simulink model "Tractive_System_model"  (R2025b)
settings: Solver=ode15s  StartTime=0  StopTime=169.89  MaxStep=1e-3  RelTol=1e-3  AbsTol=1e-6
PreLoadFcn:
  | vehicleData
undefined symbols (not defined in the file): FL, FR, RL, RR, vehicle
libraries: batteryecm_lib x281, fl_lib x86, nesl_utility x54, ee_lib x16, sdl_lib x10, SimscapeFluids_lib x3, BatteryEstimators x2, simulink x1, slpidlib x1, autolibshared x1, eePmsmFieldOrientedControl x1
(part 1 of 26)
settings Model: SimulationMode=accelerator  PacingRate=0.002200  Creator=muizz  LastModifiedBy=muizz
settings SolverCC: AutoScaleAbsTol=off  MaxConsecutiveMinStep=10000  ZeroCrossAlgorithm=Adaptive
settings DebuggingCC: AlgebraicLoopMsg=none  IgnoredZcDiagnostic=none

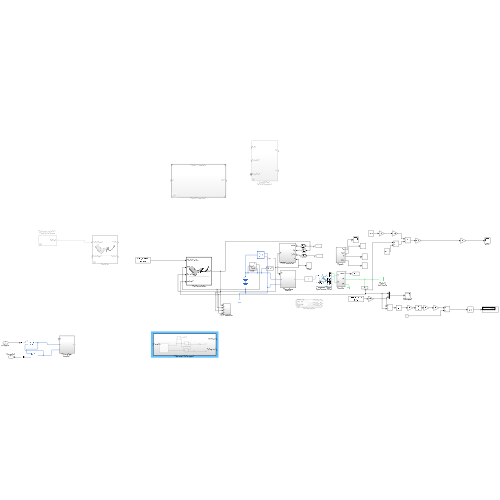
[thumbnail: Simulink's stored preview of the top-level diagram]
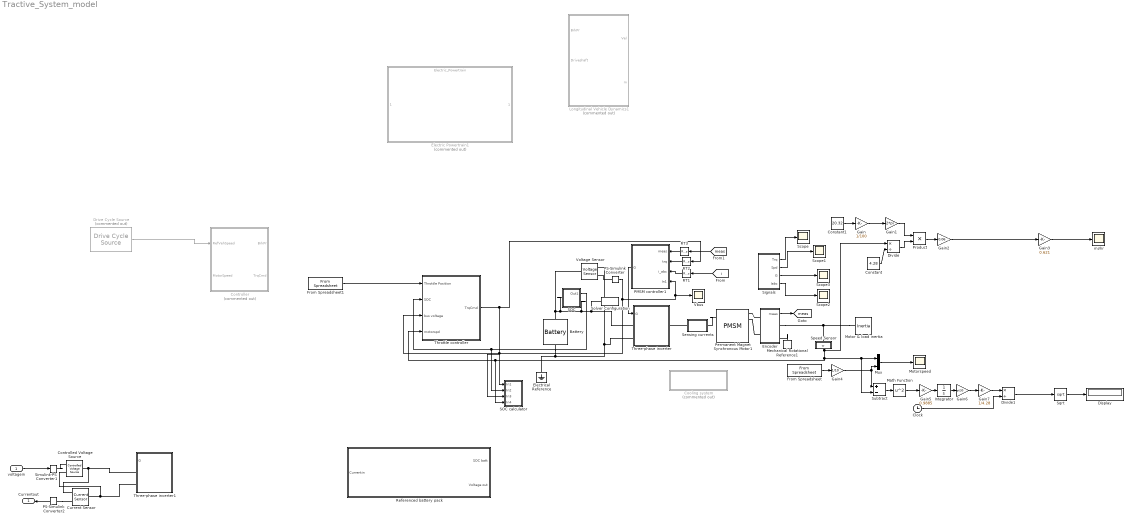
== system Tractive_System_model ==
  voltagein : Inport
  Battery : batteryecm_lib/Battery  Vnom=450 V  prm_dir=1  R1_dis=2 Ohm  R1_ch=2 Ohm  R1=0.001 Ohm  prm_AH=1  AH=14000 hr*A  V1=470 V  AH1=5000 hr*A  prm_R2=1  R2=inf Ohm  Tmeas=298.15 K  charge_measurement_port=simscape.enum.battery.enable.no  prm_dyn=1  Rp1=0.005 Ohm  tau1=30 s  Rp2=0.005 Ohm  tau2=30 s  Rp3=0.005 Ohm  tau3=30 s  Rp4=0.005 Ohm  tau4=30 s  Rp5=0.005 Ohm  tau5=30 s  prm_fade=1  N_fade=100  AH_fade=45 hr*A  R1_fade=2.02 Ohm  R1_ch_fade=2.02 Ohm  V1_fade=10.35 V  prm_age=1  prm_age_OCV=1  OCV_age=0.9  SOC_age=60  Tmeas_age=298.15 K  delta_time_age_vec=[0] d  temperature_age_vec=[273] K  OCV_scaling_age=2.2134e6  OCV_offset_age=1.632e6  temp_exp_age=0.515833569 V  t_exp_age=0.75  Vnom_T2=12 V  R1_T2=2.2 Ohm  R1_T2_dis=2.2 Ohm  R1_T2_ch=2.2 Ohm  V1_T2=11.4 V  R2_T2=2200 Ohm  Rp1_T2=0.005 Ohm  tau1_T2=30 s  Rp2_T2=0.005 Ohm  tau2_T2=30 s  Rp3_T2=0.005 Ohm  tau3_T2=30 s  Rp4_T2=0.005 Ohm  tau4_T2=30 s  Rp5_T2=0.005 Ohm  tau5_T2=30 s  Tmeas2=273.15 K  thermal_port=simscape.enum.thermaleffects.omit  thermal_mass=30000 J/K  i_specify=off  i_priority=None  i=0 A  i_nominal_specify=off  i_nominal_value=1  i_nominal_unit=A  v_specify=off  v_priority=None  v=0 V  v_nominal_specify=off  v_nominal_value=1  v_nominal_unit=V  charge_specify=on  charge_priority=High  charge=7000 hr*A  charge_nominal_specify=off  charge_nominal_value=1  charge_nominal_unit=A*hr  num_cycles_specify=off  num_cycles_priority=High  num_cycles=0  num_cycles_nominal_specify=off  num_cycles_nominal_value=1  num_cycles_nominal_unit=1  temperature_specify=off  temperature_priority=High  temperature=298.15 K  temperature_nominal_specify=off  temperature_nominal_value=1  temperature_nominal_unit=K
  Clock : Clock
  Constant : Constant  Value=4.28
  Constant1 : Constant  Value=20.32
  Controlled Voltage Source : fl_lib/Electrical/Electrical Sources/Controlled Voltage Source
  Controller : Subsystem  Commented=on  TreatAsAtomicUnit=on
      mask Display: image('Images/brakeThrottle.png'); % Use "Edit Image" on toolstrip to change.
  Cooling system : Subsystem  Commented=on
  Current Sensor : fl_lib/Electrical/Electrical Sensors/Current Sensor
  Display : Display
  Divide : Product  Inputs=*/
  Divide1 : Product  Inputs=*/
  Drive Cycle Source : autolibshared/Drive Cycle Source  Commented=on  cycleVar=Workspace variable  wsVar=fsdCycle  fileVar=cycleFTP75.mat  tfinal=""  cycleRepeat=on  outAccPort=off  outGearPort=off  gearList=No gear data  t_wot1=5  xdot_woto=0  xdot_wot1=30  t_wot2=20  xdot_wot2=0  t_wotend=30  srcUnit=m/s  outUnit=km/h  srcAccUnit=m/s/s  outAccUnit=m/s^2  dt=0  aMode=1  faultOption=off  velBnd=2  velBndUnit=mph  inUnit=m/s  timeBnd=1  failOption=off  stopSim=off  maxFaultCnt=10  maxFaultTime=2  maxTotFaultTime=15  traceOption=off  dtTrace=1  traceWindow=10  lastDCname=Custom Data Set  lastOutUnit=mph  lastDT=0  lastTB=1  lastSB=2  forceCalcBound=off
  Electric Powertrain1 : ModelReference  Commented=on  ModelNameDialog=Electric_Powertrain.slx  SimulationMode=Normal  ModelReferenceVersion=1.80
  Electrical Reference : fl_lib/Electrical/Electrical Elements/Electrical Reference
  Encoder : Subsystem
  From Spreadsheet : FromSpreadsheet  FileName=E25_Run1.xls  SheetName=RPM
  From Spreadsheet1 : FromSpreadsheet  FileName=E25_Run1.xls  SheetName=Throttle
  Gain : Gain  Gain=1/100
  Gain1 : Gain  Gain=2*pi
  Gain2 : Gain  Gain=0.06
  Gain3 : Gain  Gain=0.621
  Gain4 : Gain  Gain=1/10
  Gain5 : Gain  Gain=0.9885
  Gain6 : Gain  Gain=pi/30
  Gain7 : Gain  Gain=1/4.28
  Integrator : Integrator
  Longitudinal Vehicle Dynamics1 : Subsystem  Commented=on
  Math Function : Math  Operator=square
  Mechanical Rotational Reference1 : fl_lib/Mechanical/Rotational Elements/Mechanical Rotational Reference
  Motor & load inertia : fl_lib/Mechanical/Rotational Elements/Inertia  inertia=1.0116 kg*m^2  num_ports=foundation.enum.numPorts2.one  w_specify=on  w_priority=High  w=0 rpm  w_nominal_specify=off  w_nominal_value=1  w_nominal_unit=rad/s  t_specify=off  t_priority=High  t=0 N*m  t_nominal_specify=off  t_nominal_value=1  t_nominal_unit=N*m
  Motorspeed : Scope
      settings: ActiveDisplayYMinimum=-689.17048059754359  ActiveDisplayYMaximum=5992.5343253778938  DataLoggingVariableName=ScopeData5
  Mux : Mux  Inputs=2
  PMSM controller1 : Subsystem
  PS-Simulink Converter : nesl_utility/PS-Simulink Converter  PhysicalDomain=network_engine_domain  SubClassName=ps_output  LeftPortType=input  RightPortType=output  PseudoPeriodic=off  Frequencies=[]  VectorFormat=inherit  Unit=inherit  AffineConversion=off
  PS-Simulink Converter2 : nesl_utility/PS-Simulink Converter  PhysicalDomain=network_engine_domain  SubClassName=ps_output  LeftPortType=input  RightPortType=output  PseudoPeriodic=off  Frequencies=[]  VectorFormat=inherit  Unit=inherit  AffineConversion=off
  Permanent Magnet Synchronous Motor1 : ee_lib/Electromechanical/Permanent Magnet/PMSM  port_option=ee.enum.threePhasePort.composite  winding_type=ee.enum.statorconnection.wye  machine_param=ee.enum.pmsm.parameterization.constant  nPolePairs=10  pmflux_param=ee.enum.pmflux.fluxlinkage  pm_flux_linkage=0.04 Wb  torque_constant=0.18 N*m/A  back_emf_constant=0.18 V/(rad/s)  stator_param=ee.enum.statorparam.LdLqL0  Ld=1.25e-4 H  Lq=1.3e-4 H  idVec=[-200, 0, 200] A  iqVec=[-200, 0, 200] A  LdMatrix=0.0002 * ones(3, 3) H  LqMatrix=0.0002 * ones(3, 3) H  PmMatrix=0.1 * ones(3, 3) Wb  ktMatrix=0.18 * ones(3, 3) N*m/A  keMatrix=0.18 * ones(3, 3) V/(rad/s)  L0=L0 H  Ls=0.0002 H  Lm=0.00002 H  Ms=0.00002 H  Rs=0.012 Ohm  zero_sequence=ee.enum.park.zerosequence.exclude  axes_param=ee.enum.rotorangle.qaxis  loss_param=ee.enum.ironloss.none  losses_oc=[0, 0, 0] W  losses_sc=[0, 0, 0] W  f_losses=60 Hz  Isc_losses=95 A  J=0 kg*m^2  lam=0 N*m/(rad/s)  i_d_specify=off  i_d_priority=None  i_d=0 A  i_d_nominal_specify=off  i_d_nominal_value=1  i_d_nominal_unit=A  i_q_specify=off  i_q_priority=None  i_q=0 A  i_q_nominal_specify=off  i_q_nominal_value=1  i_q_nominal_unit=A  torque_specify=off  torque_priority=None  torque=0 N*m  torque_nominal_specify=off  torque_nominal_value=1  torque_nominal_unit=N*m  angular_velocity_specify=on  angular_velocity_priority=None  angular_velocity=0 rpm  angular_velocity_nominal_specify=off  angular_velocity_nominal_value=1  angular_velocity_nominal_unit=rpm  angular_position_specify=on  angular_position_priority=High  angular_position=0 rad  angular_position_nominal_specify=off  angular_position_nominal_value=1  angular_position_nominal_unit=deg  alpha=3.93e-3 1/K  alpha_flux=-0.001 1/K  Tmeas=298.15 K  stator_thermal_mass=100 J/K  rotor_thermal_mass=200 J/K  Rm_percent_rotor=90  Rd_percent_rotor=30  temperatureA_specify=off  temperatureA_priority=High  temperatureA=25 degC  temperatureA_nominal_specify=off  temperatureA_nominal_value=1  temperatureA_nominal_unit=degC  temperatureB_specify=off  temperatureB_priority=High  temperatureB=25 degC  temperatureB_nominal_specify=off  temperatureB_nominal_value=1  temperatureB_nominal_unit=degC  temperatureC_specify=off  temperatureC_priority=High  temperatureC=25 degC  temperatureC_nominal_specify=off  temperatureC_nominal_value=1  temperatureC_nominal_unit=degC  temperatureR_specify=off  temperatureR_priority=High  temperatureR=25 degC  temperatureR_nominal_specify=off  temperatureR_nominal_value=1  temperatureR_nominal_unit=degC
      settings: InternalSimscapePortConfiguration="{\"Bottom\":[],\"Left\":[{\"id\":\"N\",\"label\":\"~\",\"type\":\"foundation.electrical.three_phase\"},{\"id\":\"HR\",\"label\":\"HR\",\"type\":\"foundation.thermal.thermal\"}],\"Right\":[{\"id\":\"R\",\"label\":\"R\",\"type\":\"foundation.mechanical.rotational.rotational\"},{\"id\":\"C\",\"label\":\"C\",\"type\":\"foundation.mechanical.rotational.rotational\"},{\"id\":\"HA\",\"label\":\"HA\",\"type\":\"foundation.thermal.thermal\"},{\"id\":\"HB\",\"label\":\"HB\",\"type\":\"foundation.thermal.thermal\"},{\"id\":\"HC\",\"label\":\"HC\",\"type\":\"foundation.thermal.thermal\"}],\"Top\":[]}"
  Product : Product
  RT1 : RateTransition  OutPortSampleTime=1e-5
  RT2 : RateTransition  OutPortSampleTime=1e-5
  RT3 : RateTransition  OutPortSampleTime=1e-5
  "Referenced battery pack " : Subsystem  TreatAsAtomicUnit=on
  SOC : Subsystem
  SOC calculator : Subsystem
  Scope{,1..3} (4 alike) : Scope
      Scope settings: ActiveDisplayYMinimum=-50.625253953054461  ActiveDisplayYMaximum=50.62524512492179  DataLoggingVariableName=ScopeData6
      Scope1 settings: ActiveDisplayYMinimum=-1907.899738969727  ActiveDisplayYMaximum=6138.7110691558973  DataLoggingVariableName=ScopeData7
      Scope2 settings: ActiveDisplayYMinimum=-181.90652911018958  ActiveDisplayYMaximum=169.90814228402508  DataLoggingVariableName=ScopeData8
      Scope3 settings: ActiveDisplayYMinimum=-1  ActiveDisplayYMaximum=1  DataLoggingVariableName=ScopeData9
  Sensing currents : Subsystem
      mask Display: disp('i')
  "Signals " : Subsystem
  Simulink-PS Converter1 : nesl_utility/Simulink-PS Converter  PhysicalDomain=network_engine_domain  SubClassName=ps_input  LeftPortType=input  RightPortType=output  PseudoPeriodic=off  Frequencies=[]  NoiseDistribution=none  NoiseParameters=[]  Unit=1  AffineConversion=off  FilteringAndDerivatives=provide  SimscapeFilterOrder=1  InputFilterTimeConstant=0.001  UdotUserProvided=0
  Solver Configuration : nesl_utility/Solver Configuration  PhysicalDomain=network_engine_domain  SubClassName=solver  LeftPortType=input  RightPortType=generic  Tones=[]  Harmonics=[]  SimulateNoise=off  Profile=off  UseLocalSampling=off  EnableSwitchedLinearOptims=on  FrequencyDomain=off  UseCCode=off  RelTol=0.001  AbsTol=1e-06  MinStep=1e-09  ToWorkspace=off  RevertToSquareIcSolve=off  NumHomotopyIterations=100  PhasorMode=off  PhasorModeNumHarmonics=1  ConsistencySolver=NEWTON_FTOL  IndexReductionMethod=DerivativeReplacement  DoDC=off  ResidualTolerance=1e-9  ConsistencyTolSource=GLOBAL  ConsistencyAbsTol=0.001  ConsistencyRelTol=0.001  ConsistencyTolFactor=0.001  UseLocalSolver=on  LocalSolverChoice=NE_PARTITIONING_ADVANCER  ResolveIndetEquations=on  FunctionEvalNumThread=1  LocalSolverSampleTime=1e-5  DoFixedCost=off  MaxNonlinIter=4  MaxModeIter=2  ComputeImpulses=off  ImpulseIterations=2  LinearAlgebra=auto  LinearAlgebraNumThread=0  EquationFormulation=NE_TIME_EF  DelaysMemoryBudget=1024  AutomaticFiltering=on  FilteringTimeConstant=0.001  PartitionStorageMethod=AS_NEEDED  PartitionMemoryBudget=1024  PartitionMethod=FAST  MultibodyUseLocalSolver=off  MultibodyLocalSolverChoice=ODE1  MultibodyLocalSolverSampleTime=0.001
  Speed Sensor : Subsystem
      mask Display: disp('w')
  Sqrt : Sqrt
  Subtract : Sum  Inputs=+-
  Three-phase inverter : Subsystem
  Three-phase inverter1 : Subsystem
  Throttle controller : Subsystem  TreatAsAtomicUnit=on
      mask Display: image('Images/brakeThrottle.png'); % Use "Edit Image" on toolstrip to change.
  Vbus : Scope
      settings: ActiveDisplayYMinimum=403.93858192794437  ActiveDisplayYMaximum=455.46174198734315  DataLoggingVariableName=ScopeData13
  Voltage Sensor : fl_lib/Electrical/Electrical Sensors/Voltage Sensor
  mi/hr : Scope
      settings: ActiveDisplayYMinimum=-2.4921742496498496  ActiveDisplayYMaximum=69.067219320709555  DataLoggingVariableName=ScopeData4
  Currentout : Outport
  tag scope: meas=global
  wires:
  Drive Cycle Source/1 -> Controller/1(RefVehSpeed)
  "Signals "/1(Trq) -> Scope/1
  Gain/1 -> Gain1/1
  "Signals "/4(Iabc) -> Scope2/1
  "Signals "/3(G) -> Scope3/1
  "Signals "/2(Spd) -> Scope1/1
  Constant/1 -> Divide/2
  Divide/1 -> Product/2
  Constant1/1 -> Gain/1
  PS-Simulink Converter/1 -> SOC calculator/3(In3), Throttle controller/3(bus voltage), Vbus/1, PMSM controller1/4(In1)
  Speed Sensor/1(w) -> SOC calculator/4(In4), Throttle controller/4(motorspd), Mux/1, Subtract/2, Divide/1
  Gain1/1 -> Product/1
  Product/1 -> Gain2/1
  Encoder/1(meas) -> [meas]
  Gain3/1 -> mi/hr/1
  From Spreadsheet1/1 -> Throttle controller/1(Throttle Position)
  SOC/1(Out1) -> SOC calculator/2(In2), Throttle controller/2(SOC)
  Throttle controller/1(TrqCmd) -> SOC calculator/1(In1), RT2/1
  RT1/1 -> PMSM controller1/3(i_abc)
  RT3/1 -> PMSM controller1/1(meas)
  [i] -> RT1/1
  [meas] -> RT3/1
  PMSM controller1/1(G) -> Three-phase inverter/1(G)
  RT2/1 -> PMSM controller1/2(trq)
  Gain2/1 -> Gain3/1
  Mux/1 -> Motorspeed/1
  Gain4/1 -> Subtract/1, Mux/2
  From Spreadsheet/1 -> Gain4/1
  Subtract/1 -> Math Function/1
  Math Function/1 -> Gain5/1
  Divide1/1 -> Sqrt/1
  Integrator/1 -> Gain6/1
  Sqrt/1 -> Display/1
  Clock/1 -> Divide1/2
  Gain5/1 -> Integrator/1
  Gain6/1 -> Gain7/1
  Gain7/1 -> Divide1/1
  PS-Simulink Converter2/1 -> Currentout/1
  voltagein/1 -> Simulink-PS Converter1/1
  connections:
  Voltage Sensor/RConn2 -- Electrical Reference/LConn1 -- Battery/RConn1 -- Three-phase inverter/LConn2
  Motor & load inertia/LConn1 -- Encoder/RConn1 -- Speed Sensor/LConn1
  Solver Configuration/RConn1 -- SOC/RConn1 -- Voltage Sensor/LConn1 -- Battery/LConn1 -- SOC/LConn1 -- Three-phase inverter/LConn1
  Encoder/LConn1 -- Permanent Magnet Synchronous Motor1/RConn1
  PS-Simulink Converter/LConn1 -- Voltage Sensor/RConn1
  Permanent Magnet Synchronous Motor1/LConn1 -- Sensing currents/RConn1
  Encoder/LConn2 -- Permanent Magnet Synchronous Motor1/RConn2
  Sensing currents/LConn1 -- Three-phase inverter/RConn1
  Mechanical Rotational Reference1/LConn1 -- Encoder/RConn2
  Three-phase inverter1/LConn2 -- Controlled Voltage Source/RConn2 -- Current Sensor/LConn1
  Controlled Voltage Source/LConn1 -- Current Sensor/RConn2 -- Three-phase inverter1/LConn1
  PS-Simulink Converter2/LConn1 -- Current Sensor/RConn1
  Simulink-PS Converter1/RConn1 -- Controlled Voltage Source/RConn1

== system Tractive_System_model/Controller ==
  RefVehSpeed : Inport
  MotorSpeed : Inport  Port=2
  Control : Subsystem
  Motor Speed Reference : Subsystem
  Motor spd : Scope
      settings: ActiveDisplayYMinimum=-557.16498453715531  ActiveDisplayYMaximum=5014.4848608343991  DataLoggingVariableName=ScopeData3
  BrkPr : Outport
  TrqCmd : Outport  Port=2
  tag scope: Ref=global
  wires:
  RefVehSpeed/1 -> [Ref], Motor Speed Reference/1(VehSpd)
  MotorSpeed/1 -> Control/1(In1)
  Motor Speed Reference/1(MotorSpdRef) -> Motor spd/1, Control/2(Motor Speed Ref)  "Motor Speed Ref"
  Control/1(Cal Pressure) -> BrkPr/1
  Control/2(MotCmdTrq) -> TrqCmd/1  "Motor Speed"

== system Tractive_System_model/Cooling system ==
  Ambient Temperature : fl_lib/Physical Signals/Sources/PS Constant  constant=300.15 K
  "Cooling system " : Subsystem
  Subsystem1 : Subsystem
  Temperature Source : fl_lib/Thermal/Thermal Sources/Controlled Temperature Source
  Thermal Reference : fl_lib/Thermal/Thermal Elements/Thermal Reference
  Thermal model : Subsystem  Tag=PublishSubsystem
  ARMS_IN : PMIOPort  Side=Left
  VDC_IN : PMIOPort  Port=2  Side=Left
  Winding C : PMIOPort  Port=3  Side=Right
  Winding B : PMIOPort  Port=4  Side=Right
  Winding A : PMIOPort  Port=5  Side=Right
  Pressure : PMIOPort  Port=6  Side=Left
  Rotor : PMIOPort  Port=7  Side=Left
  connections:
  Subsystem1/LConn2 -- VDC_IN/RConn1
  "Cooling system "/LConn1 -- Pressure/RConn1
  Thermal model/RConn2 -- Winding B/RConn1
  Temperature Source/RConn2 -- Thermal Reference/LConn1
  Thermal model/RConn3 -- Winding A/RConn1
  Temperature Source/LConn1 -- Thermal model/LConn2
  Thermal model/LConn1 -- Rotor/RConn1 -- "Cooling system "/RConn2
  Ambient Temperature/RConn1 -- Temperature Source/RConn1
  Subsystem1/RConn1 -- "Cooling system "/RConn1
  Thermal model/RConn1 -- Winding C/RConn1
  Subsystem1/LConn1 -- ARMS_IN/RConn1

== system Tractive_System_model/Encoder ==
  Ideal Rotational Motion Sensor : fl_lib/Mechanical/Mechanical Sensors/Ideal Rotational Motion Sensor  reference=foundation.enum.MeasurementReference.difference  acceleration_port=false  velocity_port=true  position_port=true  wrap_angle=simscape.enum.onoff.off  offset=0 deg
  Ideal Torque Sensor : fl_lib/Mechanical/Mechanical Sensors/Ideal Torque Sensor
  Mux : Mux  Inputs=2
  PS-Simulink Converter : nesl_utility/PS-Simulink Converter  PhysicalDomain=network_engine_domain  SubClassName=ps_output  LeftPortType=input  RightPortType=output  PseudoPeriodic=off  Frequencies=[]  VectorFormat=1-D array  Unit=rad/s  AffineConversion=off
  PS-Simulink Converter1 : nesl_utility/PS-Simulink Converter  PhysicalDomain=network_engine_domain  SubClassName=ps_output  LeftPortType=input  RightPortType=output  PseudoPeriodic=off  Frequencies=[]  VectorFormat=1-D array  Unit=rad  AffineConversion=off
  PS-Simulink Converter2 : nesl_utility/PS-Simulink Converter  PhysicalDomain=network_engine_domain  SubClassName=ps_output  LeftPortType=input  RightPortType=output  PseudoPeriodic=off  Frequencies=[]  VectorFormat=1-D array  Unit=N*m  AffineConversion=off
  1L : PMIOPort  Side=Left
  2L : PMIOPort  Port=2  Side=Left
  1R : PMIOPort  Port=3  Side=Right
  2R : PMIOPort  Port=4  Side=Right
  meas : Outport  VectorParamsAs1DForOutWhenUnconnected=off
  tag scope: trqMotor=global, wMotor=global
  wires:
  PS-Simulink Converter2/1 -> [trqMotor]
  Mux/1 -> meas/1
  PS-Simulink Converter1/1 -> Mux/2
  PS-Simulink Converter/1 -> [wMotor], Mux/1
  connections:
  Ideal Torque Sensor/RConn2 -- PS-Simulink Converter2/LConn1
  1L/RConn1 -- Ideal Torque Sensor/LConn1
  2R/RConn1 -- 2L/RConn1 -- Ideal Rotational Motion Sensor/RConn1
  Ideal Rotational Motion Sensor/LConn1 -- 1R/RConn1 -- Ideal Torque Sensor/RConn1
  Ideal Rotational Motion Sensor/RConn2 -- PS-Simulink Converter/LConn1
  Ideal Rotational Motion Sensor/RConn3 -- PS-Simulink Converter1/LConn1

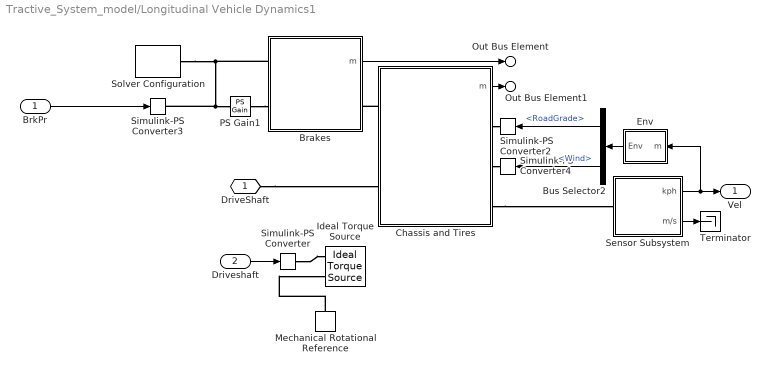
== system Tractive_System_model/Longitudinal Vehicle Dynamics1 ==
  BrkPr : Inport
  Driveshaft : Inport  Port=2
  Brakes : Subsystem
  Bus Selector2 : BusSelector  OutputSignals=RoadGrade,Wind
  Chassis and Tires : Subsystem
  Env : Subsystem
  Ideal Torque Source : fl_lib/Mechanical/Mechanical Sources/Ideal Torque Source
  Mechanical Rotational Reference : fl_lib/Mechanical/Rotational Elements/Mechanical Rotational Reference
  PS Gain1 : fl_lib/Physical Signals/Functions/PS Gain  gain=1
  Sensor Subsystem : Subsystem
  Simulink-PS Converter : nesl_utility/Simulink-PS Converter  PhysicalDomain=network_engine_domain  SubClassName=ps_input  LeftPortType=input  RightPortType=output  PseudoPeriodic=off  Frequencies=[]  NoiseDistribution=none  NoiseParameters=[]  Unit=N*m  AffineConversion=off  FilteringAndDerivatives=provide  SimscapeFilterOrder=1  InputFilterTimeConstant=0.001  UdotUserProvided=0
  Simulink-PS Converter2 : nesl_utility/Simulink-PS Converter  PhysicalDomain=network_engine_domain  SubClassName=ps_input  LeftPortType=input  RightPortType=output  PseudoPeriodic=off  Frequencies=[]  NoiseDistribution=none  NoiseParameters=[]  Unit=rad  AffineConversion=off  FilteringAndDerivatives=provide  SimscapeFilterOrder=1  InputFilterTimeConstant=0.001  UdotUserProvided=0
  Simulink-PS Converter3 : nesl_utility/Simulink-PS Converter  PhysicalDomain=network_engine_domain  SubClassName=ps_input  LeftPortType=input  RightPortType=output  PseudoPeriodic=off  Frequencies=[]  NoiseDistribution=none  NoiseParameters=[]  Unit=N/m^2  AffineConversion=off  FilteringAndDerivatives=provide  SimscapeFilterOrder=1  InputFilterTimeConstant=0.001  UdotUserProvided=0
  Simulink-PS Converter4 : nesl_utility/Simulink-PS Converter  PhysicalDomain=network_engine_domain  SubClassName=ps_input  LeftPortType=input  RightPortType=output  PseudoPeriodic=off  Frequencies=[]  NoiseDistribution=none  NoiseParameters=[]  Unit=m/s  AffineConversion=off  FilteringAndDerivatives=provide  SimscapeFilterOrder=1  InputFilterTimeConstant=0.001  UdotUserProvided=0
  Solver Configuration : nesl_utility/Solver Configuration  PhysicalDomain=network_engine_domain  SubClassName=solver  LeftPortType=input  RightPortType=generic  Tones=[]  Harmonics=[]  SimulateNoise=off  Profile=off  UseLocalSampling=off  EnableSwitchedLinearOptims=on  FrequencyDomain=off  UseCCode=off  RelTol=0.001  AbsTol=0.001  MinStep=1e-09  ToWorkspace=off  RevertToSquareIcSolve=off  NumHomotopyIterations=100  PhasorMode=off  PhasorModeNumHarmonics=1  ConsistencySolver=NEWTON_XTOL_AFTER_FTOL  IndexReductionMethod=DerivativeReplacement  DoDC=off  ResidualTolerance=1e-09  ConsistencyTolSource=GLOBAL  ConsistencyAbsTol=0.001  ConsistencyRelTol=0.001  ConsistencyTolFactor=0.001  UseLocalSolver=on  LocalSolverChoice=NE_BACKWARD_EULER_ADVANCER  ResolveIndetEquations=on  FunctionEvalNumThread=1  LocalSolverSampleTime=1e-4  DoFixedCost=off  MaxNonlinIter=3  MaxModeIter=2  ComputeImpulses=off  ImpulseIterations=2  LinearAlgebra=auto  LinearAlgebraNumThread=0  EquationFormulation=NE_TIME_EF  DelaysMemoryBudget=1024  AutomaticFiltering=on  FilteringTimeConstant=0.001  PartitionStorageMethod=AS_NEEDED  PartitionMemoryBudget=1024  PartitionMethod=ROBUST  MultibodyUseLocalSolver=off  MultibodyLocalSolverChoice=ODE1  MultibodyLocalSolverSampleTime=0.001
  Terminator : Terminator
  DriveShaft : PMIOPort  Side=Left
  Vel : Outport
  Out Bus Element : Outport  Port=2  PortName=m  Element=Brakes
  Out Bus Element1 : Outport  Port=2  PortName=m  Element=Chassis
  wires:
  Sensor Subsystem/1(kph) -> Vel/1, Env/1(m)
  Env/1(Env) -> Bus Selector2/1
  Bus Selector2/1 -> Simulink-PS Converter2/1  "<RoadGrade>"
  Bus Selector2/2 -> Simulink-PS Converter4/1  "<Wind>"
  BrkPr/1 -> Simulink-PS Converter3/1
  Sensor Subsystem/2(m/s) -> Terminator/1
  Brakes/1(m) -> Out Bus Element/1
  Chassis and Tires/1(m) -> Out Bus Element1/1
  Driveshaft/1 -> Simulink-PS Converter/1
  connections:
  Brakes/LConn1 -- Solver Configuration/RConn1 -- Simulink-PS Converter3/RConn1 -- PS Gain1/LConn1
  Chassis and Tires/RConn1 -- Simulink-PS Converter2/RConn1
  Chassis and Tires/RConn2 -- Simulink-PS Converter4/RConn1
  Chassis and Tires/LConn1 -- Brakes/RConn1
  Chassis and Tires/RConn3 -- Sensor Subsystem/LConn1
  PS Gain1/RConn1 -- Brakes/LConn2
  DriveShaft/RConn1 -- Chassis and Tires/LConn2
  Mechanical Rotational Reference/LConn1 -- Ideal Torque Source/RConn2
  Simulink-PS Converter/RConn1 -- Ideal Torque Source/RConn1

== system Tractive_System_model/PMSM controller1 ==
  meas : Inport
  trq : Inport  Port=2
  i_abc : Inport  Port=3
  In1 : Inport  Port=4
  Bus Selector : BusSelector  OutputSignals=iabc [A],Reference,TqRef [N*m]
  Demux1 : Demux  Outputs=2
  PMSM Field-Oriented Control : eePmsmFieldOrientedControl/PMSM Field-Oriented Control  winding_type=Wye-wound  CtrlMode=Torque control  Vnom=600  Pmax=80000  Tmax=150  p=10  Vdc_on=10  Ts=1e-5  Tsc=Tsc  CtrlType=PI control  Kp_w=60  Ki_w=300*2  Kv_w=1  Kaw_w=1000  RefType=Zero d-axis control  rpmVec=[0, 3000]  TqVec=[-100, 0, 100]  VdcVec=[300, 350]  PWMMode=SPWM: sinusoidal PWM  ModFactor=1  idMatrix=zeros(2,3,2)  iqMatrix=zeros(2,3,2)  psim=0.04  Ld=0.00024  Lq=0.00029  Rs=0.01  AxisAlignment=Q-axis  Kp_id=0.7854  Ki_id=75.4  Kaw_id=1000  Kp_iq=0.8168  Ki_iq=75.40  Kaw_iq=1000  AxisPrio=Q-axis  ActZC=off  ActFF=on  ParamTypeFF=Constant parameters  LdFF=1.25e-4  LqFF=1.3e-4  psimFF=0.04  idVect=[-200, 0, 200]  iqVect=[-200, 0, 200]  LdMatrix=0.0002 * ones(3, 3)  LqMatrix=0.0002 * ones(3, 3)  psimMatrix=0.04 * ones(3, 3)  CPWMMode=SPWM: sinusoidal PWM  fsw=10000
  G : Outport  VectorParamsAs1DForOutWhenUnconnected=off
  tag scope: G=global, iMotor=global, trqDemand=global, wDemand=global
  wires:
  PMSM Field-Oriented Control/1 -> G/1, [G]
  In1/1 -> PMSM Field-Oriented Control/5
  PMSM Field-Oriented Control/2 -> Bus Selector/1
  i_abc/1 -> PMSM Field-Oriented Control/2
  meas/1 -> Demux1/1
  Demux1/1 -> PMSM Field-Oriented Control/3
  Demux1/2 -> PMSM Field-Oriented Control/4
  Bus Selector/1 -> [iMotor]  "<iabc [A]>"
  Bus Selector/2 -> [wDemand]  "<Reference>"
  Bus Selector/3 -> [trqDemand]  "<TqRef [N*m]>"
  trq/1 -> PMSM Field-Oriented Control/1

== system Tractive_System_model/Referenced battery pack  ==
  Currentin : Inport
  Accumalator : Subsystem
  Controlled Current Source : fl_lib/Electrical/Electrical Sources/Controlled Current Source
  PS-Simulink Converter1 : nesl_utility/PS-Simulink Converter  PhysicalDomain=network_engine_domain  SubClassName=ps_output  LeftPortType=input  RightPortType=output  PseudoPeriodic=off  Frequencies=[]  VectorFormat=inherit  Unit=inherit  AffineConversion=off
  SOC1 : Subsystem
  Simulink-PS Converter : nesl_utility/Simulink-PS Converter  PhysicalDomain=network_engine_domain  SubClassName=ps_input  LeftPortType=input  RightPortType=output  PseudoPeriodic=off  Frequencies=[]  NoiseDistribution=none  NoiseParameters=[]  Unit=1  AffineConversion=off  FilteringAndDerivatives=provide  SimscapeFilterOrder=1  InputFilterTimeConstant=0.001  UdotUserProvided=0
  Voltage Sensor1 : fl_lib/Electrical/Electrical Sensors/Voltage Sensor
  SOC batt : Outport
  Voltage out : Outport  Port=2
  wires:
  Currentin/1 -> Simulink-PS Converter/1
  PS-Simulink Converter1/1 -> Voltage out/1
  SOC1/1(SOC batt) -> SOC batt/1
  connections:
  Controlled Current Source/LConn1 -- SOC1/LConn1 -- Accumalator/LConn1 -- SOC1/RConn1 -- Voltage Sensor1/RConn2
  PS-Simulink Converter1/LConn1 -- Voltage Sensor1/RConn1
  Accumalator/LConn2 -- Controlled Current Source/RConn2 -- Voltage Sensor1/LConn1
  Simulink-PS Converter/RConn1 -- Controlled Current Source/RConn1

== system Tractive_System_model/SOC ==
  Constant2 : Constant
  Current Sensor : fl_lib/Electrical/Electrical Sensors/Current Sensor
  PS-Simulink Converter1 : nesl_utility/PS-Simulink Converter  PhysicalDomain=network_engine_domain  SubClassName=ps_output  LeftPortType=input  RightPortType=output  PseudoPeriodic=off  Frequencies=[]  VectorFormat=inherit  Unit=inherit  AffineConversion=off
  SOC : Scope
      settings: ActiveDisplayYMinimum=-1  ActiveDisplayYMaximum=1  DataLoggingVariableName=ScopeData12
  SOC Estimator (Coulomb Counting) : BatteryEstimators/SOC Estimator (Coulomb Counting)  CurrentInputPartition=on  AH=27  Ts=1  DataType=Inherit: auto
      settings: LibrarySourceBlock=|
      | batt_sl_lib/Estimators/SOC Estimator
      | (Coulomb Counting)
  Conn1 : PMIOPort  Side=Left
  Conn2 : PMIOPort  Port=2  Side=Right
  Out1 : Outport
  wires:
  Constant2/1 -> SOC Estimator (Coulomb Counting)/2
  SOC Estimator (Coulomb Counting)/1 -> SOC/1, Out1/1  "Coulomb counting"
  PS-Simulink Converter1/1 -> SOC Estimator (Coulomb Counting)/1
  connections:
  Current Sensor/LConn1 -- Conn1/RConn1
  Current Sensor/RConn2 -- Conn2/RConn1
  PS-Simulink Converter1/LConn1 -- Current Sensor/RConn1

== system Tractive_System_model/SOC calculator ==
  In1 : Inport
  In2 : Inport  Port=2
  In3 : Inport  Port=3
  In4 : Inport  Port=4
  Divide1 : Product  Inputs=*/
  Gain4 : Gain  Gain=pi/30
  Gain5 : Gain  Gain=0.9
  Gain6 : Gain  Gain=1/18000
  Integrator : Integrator
  Product1 : Product
  SOC Return : Scope
      settings: ActiveDisplayYMinimum=-1.0236940402923616  ActiveDisplayYMaximum=-0.7867536373688393  DataLoggingVariableName=ScopeData14
  Sum : Sum  Inputs=|+-
  wires:
  In3/1 -> Divide1/2
  In1/1 -> Product1/1
  Gain4/1 -> Product1/2
  Integrator/1 -> Gain6/1
  In2/1 -> Sum/2
  Divide1/1 -> Integrator/1
  Gain6/1 -> Sum/1
  In4/1 -> Gain4/1
  Gain5/1 -> Divide1/1
  Sum/1 -> SOC Return/1
  Product1/1 -> Gain5/1

== system Tractive_System_model/Sensing currents ==
  Current Sensor : ee_lib/Sensors & Transducers/Current Sensor (Three-Phase)
  Gain : Gain  Commented=through  Gain=1/sqrt(3)
  PS-Simulink Converter : nesl_utility/PS-Simulink Converter  PhysicalDomain=network_engine_domain  SubClassName=ps_output  LeftPortType=input  RightPortType=output  PseudoPeriodic=off  Frequencies=[]  VectorFormat=1-D array  Unit=A  AffineConversion=off
  Conn1 : PMIOPort  Side=Left
  Conn2 : PMIOPort  Port=2  Side=Right
  tag scope: i=global
  wires:
  PS-Simulink Converter/1 -> Gain/1
  Gain/1 -> [i]
  connections:
  Current Sensor/RConn1 -- PS-Simulink Converter/LConn1
  Conn2/RConn1 -- Current Sensor/RConn2
  Current Sensor/LConn1 -- Conn1/RConn1

== system Tractive_System_model/Signals  ==
  Mux : Mux  Inputs=2
  Mux1 : Mux  Inputs=2
  RT{1..4} (4 alike) : RateTransition  OutPortSampleTime=1e-5
  rad/s2rpm : Gain  Gain=60/(2*pi)
  Trq : Outport  VectorParamsAs1DForOutWhenUnconnected=off
  Spd : Outport  Port=2  VectorParamsAs1DForOutWhenUnconnected=off
  G : Outport  Port=3  VectorParamsAs1DForOutWhenUnconnected=off
  Iabc : Outport  Port=4  VectorParamsAs1DForOutWhenUnconnected=off
  wires:
  [trqDemand] -> Mux/1
  [G] -> G/1  "Gates"
  Mux1/1 -> rad/s2rpm/1
  Mux/1 -> RT1/1  "Torque"
  [iMotor] -> RT3/1  "Currents"
  [wDemand] -> Mux1/1
  rad/s2rpm/1 -> RT2/1  "Speed"
  [trqMotor] -> RT4/1
  RT1/1 -> Trq/1  "Torque"
  RT2/1 -> Spd/1  "Speed"
  RT3/1 -> Iabc/1  "Currents"
  RT4/1 -> Mux/2
  [wMotor] -> Mux1/2

== system Tractive_System_model/Speed Sensor ==
  Mechanical Rotational Reference1 : fl_lib/Mechanical/Rotational Elements/Mechanical Rotational Reference
  Motion Sensor : fl_lib/Mechanical/Mechanical Sensors/Ideal Rotational Motion Sensor  reference=foundation.enum.MeasurementReference.difference  acceleration_port=false  velocity_port=true  position_port=true  wrap_angle=simscape.enum.onoff.off  offset=0 rad
  PS Terminator : fl_lib/Physical Signals/Sinks/PS Terminator
  PS-Simulink Converter 2 : nesl_utility/PS-Simulink Converter  PhysicalDomain=network_engine_domain  SubClassName=ps_output  LeftPortType=input  RightPortType=output  PseudoPeriodic=off  Frequencies=[]  VectorFormat=1-D array  Unit=rpm  AffineConversion=off
  R : PMIOPort  Side=Left
  w : Outport
  wires:
  PS-Simulink Converter 2/1 -> w/1
  connections:
  Motion Sensor/LConn1 -- R/RConn1
  Motion Sensor/RConn3 -- PS Terminator/LConn1
  Motion Sensor/RConn1 -- Mechanical Rotational Reference1/LConn1
  Motion Sensor/RConn2 -- PS-Simulink Converter 2/LConn1
